simulink model "Model"  (R2024b)
settings: Solver=ode45  StartTime=0.0  StopTime=10.0  MaxStep=Ts  RelTol=1e-3
InitFcn:
  | clear
  | run('../../utils/params.m')
undefined symbols (not defined in the file): body, drv, Fv1, g, gbox, M11, M22, mot, ms22g, sens, Ts, ua2tau, wheel
libraries: simulink_extras x5
settings Model: Creator=Banaan  LastModifiedBy=Banaan

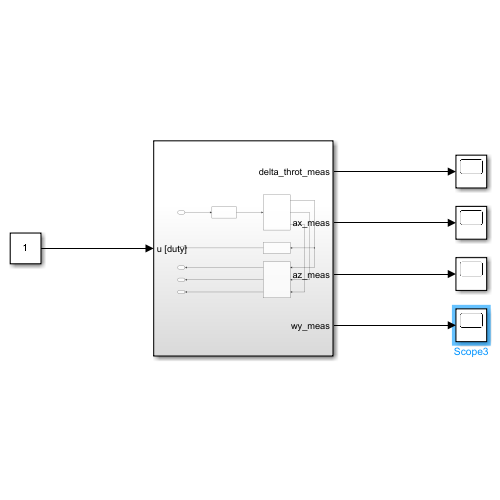
[thumbnail: Simulink's stored preview of the top-level diagram]
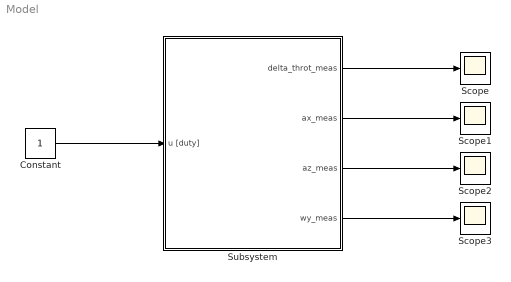
== system Model ==
  Constant : Constant
  Scope{,1..3} (4 alike) : Scope
  Subsystem : Subsystem
  wires:
  Constant/1 -> Subsystem/1(u [duty])
  Subsystem/1(delta_throt_meas) -> Scope/1
  Subsystem/2(ax_meas) -> Scope1/1
  Subsystem/3(az_meas) -> Scope2/1
  Subsystem/4(wy_meas) -> Scope3/1

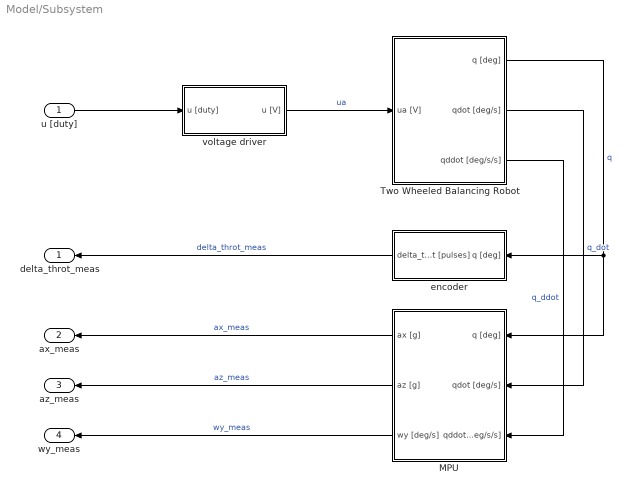
== system Model/Subsystem ==
  u [duty] : Inport
  MPU : Subsystem
  Two Wheeled Balancing Robot : Subsystem
  encoder : Subsystem
  voltage driver : Subsystem
  delta_throt_meas : Outport
  ax_meas : Outport  Port=2
  az_meas : Outport  Port=3
  wy_meas : Outport  Port=4
  wires:
  Two Wheeled Balancing Robot/1(q [deg]) -> encoder/1(q [deg]), MPU/1(q [deg])  "q"
  MPU/3(wy [deg/s]) -> wy_meas/1  "wy_meas"
  encoder/1(delta_throt [pulses]) -> delta_throt_meas/1  "delta_throt_meas"
  MPU/2(az [g]) -> az_meas/1  "az_meas"
  voltage driver/1(u [V]) -> Two Wheeled Balancing Robot/1(ua [V])  "ua"
  Two Wheeled Balancing Robot/2(qdot [deg/s]) -> MPU/2(qdot [deg/s])  "q_dot"
  Two Wheeled Balancing Robot/3(qddot [deg/s/s]) -> MPU/3(qddot [deg/s/s])  "q_ddot"
  MPU/1(ax [g]) -> ax_meas/1  "ax_meas"
  u [duty]/1 -> voltage driver/1(u [duty])

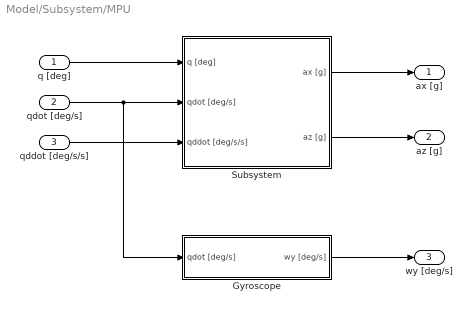
== system Model/Subsystem/MPU ==
  q [deg] : Inport
  qdot [deg/s] : Inport  Port=2
  qddot [deg/s/s] : Inport  Port=3
  Gyroscope : Subsystem
  Subsystem : Subsystem
  ax [g] : Outport
  az [g] : Outport  Port=2
  wy [deg/s] : Outport  Port=3
  wires:
  qddot [deg/s/s]/1 -> Subsystem/3(qddot [deg/s/s])
  qdot [deg/s]/1 -> Subsystem/2(qdot [deg/s]), Gyroscope/1(qdot [deg/s])
  Subsystem/2(az [g]) -> az [g]/1
  q [deg]/1 -> Subsystem/1(q [deg])
  Gyroscope/1(wy [deg/s]) -> wy [deg/s]/1
  Subsystem/1(ax [g]) -> ax [g]/1

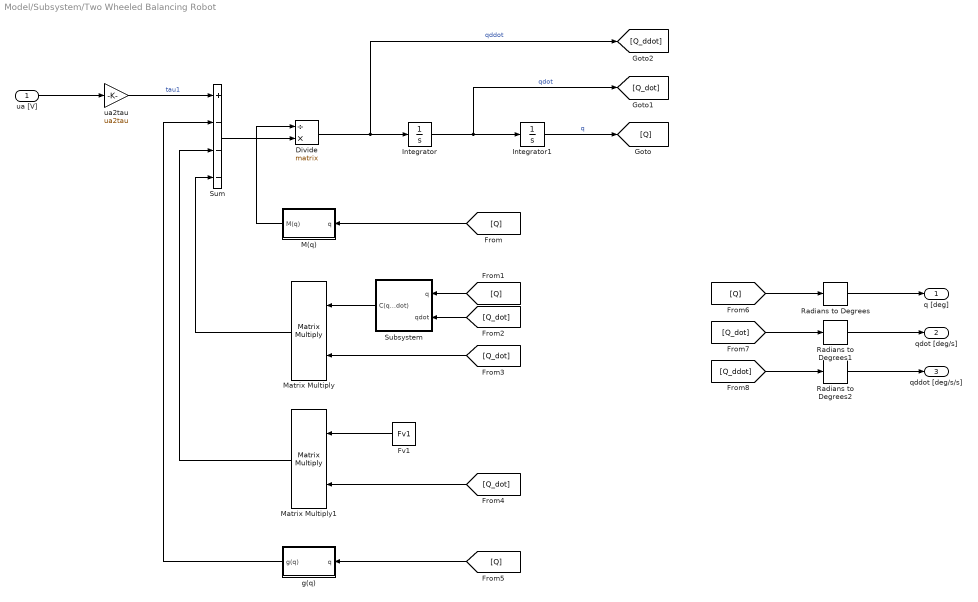
== system Model/Subsystem/Two Wheeled Balancing Robot ==
  ua [V] : Inport
  Divide : Product  Inputs=/*  Multiplication=Matrix(*)
  Fv1 : Constant  Value=Fv1
  Integrator : Integrator
  Integrator1 : Integrator
  M(q) : Subsystem
  Matrix Multiply : Product  Multiplication=Matrix(*)
  Matrix Multiply1 : Product  Multiplication=Matrix(*)
  Radians to Degrees : simulink_extras/Transformations/Radians to Degrees
  Radians to Degrees1 : simulink_extras/Transformations/Radians to Degrees
  Radians to Degrees2 : simulink_extras/Transformations/Radians to Degrees
  Subsystem : Subsystem
  Sum : Sum  Inputs=+---
  g(q) : Subsystem
  ua2tau : Gain  Gain=ua2tau
  q [deg] : Outport
  qdot [deg/s] : Outport  Port=2
  qddot [deg/s/s] : Outport  Port=3
  wires:
  [Q] -> M(q)/1(q)
  [Q_ddot] -> Radians to Degrees2/1
  Divide/1 -> [Q_ddot], Integrator/1  "qddot"
  Sum/1 -> Divide/2
  M(q)/1(M(q)) -> Divide/1
  [Q] -> Radians to Degrees/1
  Subsystem/1("C(q, qdot)") -> Matrix Multiply/1
  [Q_dot] -> Matrix Multiply1/2
  [Q_dot] -> Radians to Degrees1/1
  Matrix Multiply/1 -> Sum/4
  Integrator/1 -> [Q_dot], Integrator1/1  "qdot"
  [Q] -> Subsystem/1(q)
  Matrix Multiply1/1 -> Sum/3
  g(q)/1(g(q)) -> Sum/2
  Integrator1/1 -> [Q]  "q"
  [Q_dot] -> Subsystem/2(qdot)
  Fv1/1 -> Matrix Multiply1/1
  [Q_dot] -> Matrix Multiply/2
  ua2tau/1 -> Sum/1  "tau1"
  Radians to Degrees1/1 -> qdot [deg/s]/1
  Radians to Degrees/1 -> q [deg]/1
  [Q] -> g(q)/1(q)
  Radians to Degrees2/1 -> qddot [deg/s/s]/1
  ua [V]/1 -> ua2tau/1

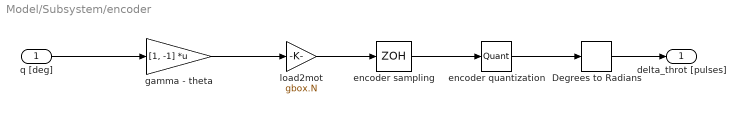
== system Model/Subsystem/encoder ==
  q [deg] : Inport
  Degrees to Radians : simulink_extras/Transformations/Degrees to Radians
  encoder quantization : Quantizer  QuantizationInterval=sens.enc.pulse2deg
  encoder sampling : ZeroOrderHold  SampleTime=Ts
  gamma - theta : Gain  Gain=[1, -1]  Multiplication=Matrix(K*u)
  load2mot : Gain  Gain=gbox.N
  delta_throt [pulses] : Outport
  wires:
  encoder sampling/1 -> encoder quantization/1
  q [deg]/1 -> gamma - theta/1
  encoder quantization/1 -> Degrees to Radians/1
  load2mot/1 -> encoder sampling/1
  gamma - theta/1 -> load2mot/1
  Degrees to Radians/1 -> delta_throt [pulses]/1

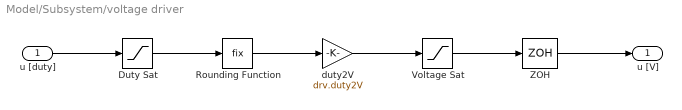
== system Model/Subsystem/voltage driver ==
  u [duty] : Inport
  Duty Sat : Saturate  UpperLimit=drv.dutymax  LowerLimit=-drv.dutymax
  Rounding Function : Rounding  Operator=fix
  Voltage Sat : Saturate  UpperLimit=drv.Vbus  LowerLimit=-drv.Vbus
  ZOH : ZeroOrderHold  SampleTime=Ts
  duty2V : Gain  Gain=drv.duty2V
  u [V] : Outport
  wires:
  Duty Sat/1 -> Rounding Function/1
  duty2V/1 -> Voltage Sat/1
  u [duty]/1 -> Duty Sat/1
  Voltage Sat/1 -> ZOH/1
  Rounding Function/1 -> duty2V/1
  ZOH/1 -> u [V]/1

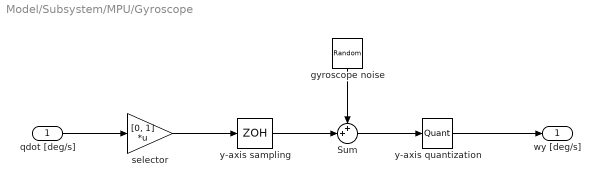
== system Model/Subsystem/MPU/Gyroscope ==
  qdot [deg/s] : Inport
  Sum : Sum  Inputs=++|
  gyroscope noise : RandomNumber  Variance=sens.mpu.gyro.noisevar  SampleTime=Ts
  selector : Gain  Gain=[0, 1]  Multiplication=Matrix(K*u)
  y-axis quantization : Quantizer  QuantizationInterval=sens.mpu.gyro.LSB2degs
  y-axis sampling : ZeroOrderHold  SampleTime=Ts
  wy [deg/s] : Outport
  wires:
  y-axis quantization/1 -> wy [deg/s]/1
  selector/1 -> y-axis sampling/1
  Sum/1 -> y-axis quantization/1
  gyroscope noise/1 -> Sum/1
  y-axis sampling/1 -> Sum/2
  qdot [deg/s]/1 -> selector/1

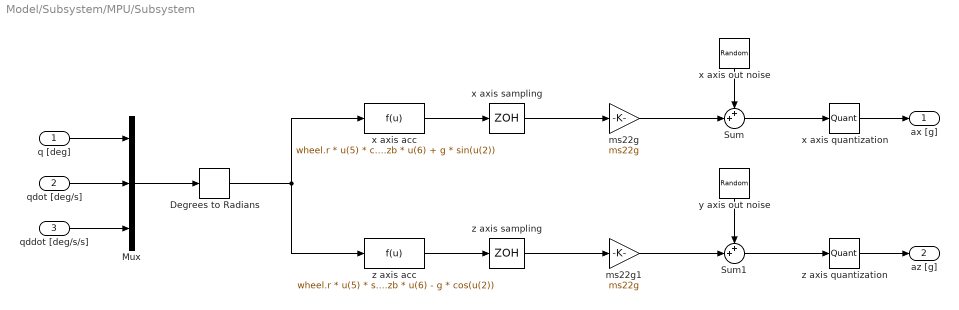
== system Model/Subsystem/MPU/Subsystem ==
  q [deg] : Inport
  qdot [deg/s] : Inport  Port=2
  qddot [deg/s/s] : Inport  Port=3
  Degrees to Radians : simulink_extras/Transformations/Degrees to Radians
  Mux : Mux  Inputs=3
  Sum : Sum  Inputs=++|
  Sum1 : Sum  Inputs=++|
  ms22g : Gain  Gain=ms22g
  ms22g1 : Gain  Gain=ms22g
  x axis out noise : RandomNumber  Variance=sens.mpu.acc.noisevar  SampleTime=Ts
  x axis quantization : Quantizer  QuantizationInterval=sens.mpu.acc.LSB2g
  x axis sampling : ZeroOrderHold  SampleTime=Ts
  x axis acc : Fcn  Expr=wheel.r * u(5) * cos(u(2)) + sens.mpu.zb * u(6) + g * sin(u(2))
  y axis out noise : RandomNumber  Variance=sens.mpu.acc.noisevar  SampleTime=Ts
  z axis quantization : Quantizer  QuantizationInterval=sens.mpu.acc.LSB2g
  z axis sampling : ZeroOrderHold  SampleTime=Ts
  z axis acc : Fcn  Expr=wheel.r * u(5) * sin(u(2)) - sens.mpu.zb * u(6) - g * cos(u(2))
  ax [g] : Outport
  az [g] : Outport  Port=2
  wires:
  x axis acc/1 -> x axis sampling/1
  z axis acc/1 -> z axis sampling/1
  x axis out noise/1 -> Sum/1
  x axis quantization/1 -> ax [g]/1
  y axis out noise/1 -> Sum1/1
  ms22g/1 -> Sum/2
  x axis sampling/1 -> ms22g/1
  ms22g1/1 -> Sum1/2
  Sum1/1 -> z axis quantization/1
  z axis sampling/1 -> ms22g1/1
  Sum/1 -> x axis quantization/1
  qdot [deg/s]/1 -> Mux/2
  z axis quantization/1 -> az [g]/1
  q [deg]/1 -> Mux/1
  qddot [deg/s/s]/1 -> Mux/3
  Mux/1 -> Degrees to Radians/1
  Degrees to Radians/1 -> z axis acc/1, x axis acc/1

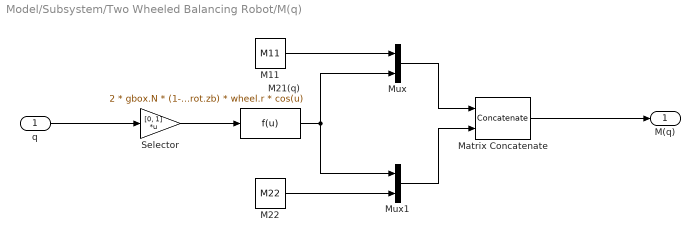
== system Model/Subsystem/Two Wheeled Balancing Robot/M(q) ==
  q : Inport
  M11 : Constant  Value=M11
  M21(q) : Fcn  Expr=2 * gbox.N * (1-gbox.N) * mot.rot.Iyy + (body.m * body.zb + 2 * mot.rot.m * mot.rot.zb) * wheel.r * cos(u)
  M22 : Constant  Value=M22
  Matrix Concatenate : Concatenate  Mode=Multidimensional array  ConcatenateDimension=2
  Mux : Mux  Inputs=2
  Mux1 : Mux  Inputs=2
  Selector : Gain  Gain=[0, 1]  Multiplication=Matrix(K*u)
  M(q) : Outport
  wires:
  M22/1 -> Mux1/2
  Selector/1 -> M21(q)/1
  M21(q)/1 -> Mux1/1, Mux/2
  Mux/1 -> Matrix Concatenate/1
  M11/1 -> Mux/1
  Matrix Concatenate/1 -> M(q)/1
  Mux1/1 -> Matrix Concatenate/2
  q/1 -> Selector/1

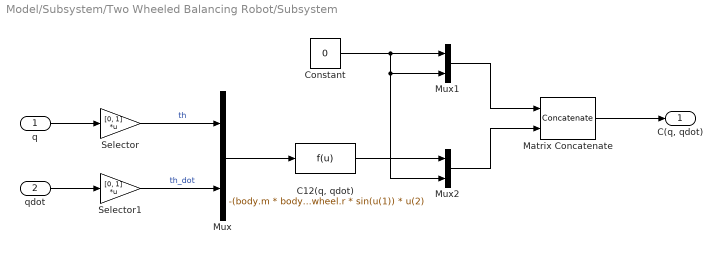
== system Model/Subsystem/Two Wheeled Balancing Robot/Subsystem ==
  q : Inport
  qdot : Inport  Port=2
  "C12(q, qdot)" : Fcn  Expr=-(body.m * body.zb + 2 * mot.rot.m * mot.rot.zb) * wheel.r * sin(u(1)) * u(2)
  Constant : Constant  Value=0
  Matrix Concatenate : Concatenate  Mode=Multidimensional array  ConcatenateDimension=2
  Mux : Mux  Inputs=2
  Mux1 : Mux  Inputs=2
  Mux2 : Mux  Inputs=2
  Selector : Gain  Gain=[0, 1]  Multiplication=Matrix(K*u)
  Selector1 : Gain  Gain=[0, 1]  Multiplication=Matrix(K*u)
  "C(q, qdot)" : Outport
  wires:
  "C12(q, qdot)"/1 -> Mux2/1
  Mux1/1 -> Matrix Concatenate/1
  Constant/1 -> Mux2/2, Mux1/2, Mux1/1
  Matrix Concatenate/1 -> "C(q, qdot)"/1
  Selector1/1 -> Mux/2  "th_dot"
  Selector/1 -> Mux/1  "th"
  Mux/1 -> "C12(q, qdot)"/1
  Mux2/1 -> Matrix Concatenate/2
  q/1 -> Selector/1
  qdot/1 -> Selector1/1

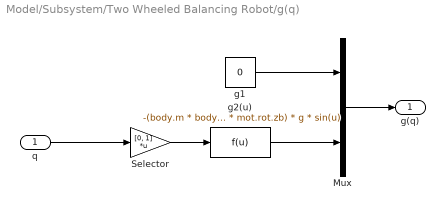
== system Model/Subsystem/Two Wheeled Balancing Robot/g(q) ==
  q : Inport
  Mux : Mux  Inputs=2
  Selector : Gain  Gain=[0, 1]  Multiplication=Matrix(K*u)
  g1 : Constant  Value=0
  g2(u) : Fcn  Expr=-(body.m * body.zb + 2 * mot.rot.m * mot.rot.zb) * g * sin(u)
  g(q) : Outport
  wires:
  Selector/1 -> g2(u)/1
  g2(u)/1 -> Mux/2
  g1/1 -> Mux/1
  q/1 -> Selector/1
  Mux/1 -> g(q)/1
